simulink model "BmrTests"  (R2020a)
settings: Solver=FixedStepDiscrete  StartTime=0.0  StopTime=inf  FixedStep=Ts  RelTol=1e-3  EnableMultiTasking=on
undefined symbols (not defined in the file): BMR, DiscIntNeverNeededParam, MSR_REQUEST
libraries: simulink x2
settings Model: Creator=tbria  LastModifiedBy=Harjot
settings OptimizationCC: LifeSpan=inf
settings DebuggingCC: SFUnexpectedBacktrackingDiag=warning  SFNoUnconditionalDefaultTransitionDiag=warning  SFExecutionAtInitializationDiag=none  ArithmeticOperatorsInVariantConditions=warning
settings SFSimCC: SimUseLocalCustomCode=off  CustomCodeUndefinedFunction=UseInterfaceOnly
settings RTWCC: RTWUseLocalCustomCode=off
settings CodeAppCC: StateflowObjectComments=on
settings GRTTargetCC: TargetLangStandard=C89/C90 (ANSI)
settings ConfigComp: CovMetricSettings=dw  CovHtmlReporting=on  CovSaveCumulativeToWorkspaceVar=on  CovSaveSingleToWorkspaceVar=on  CovExternalEMLEnable=off

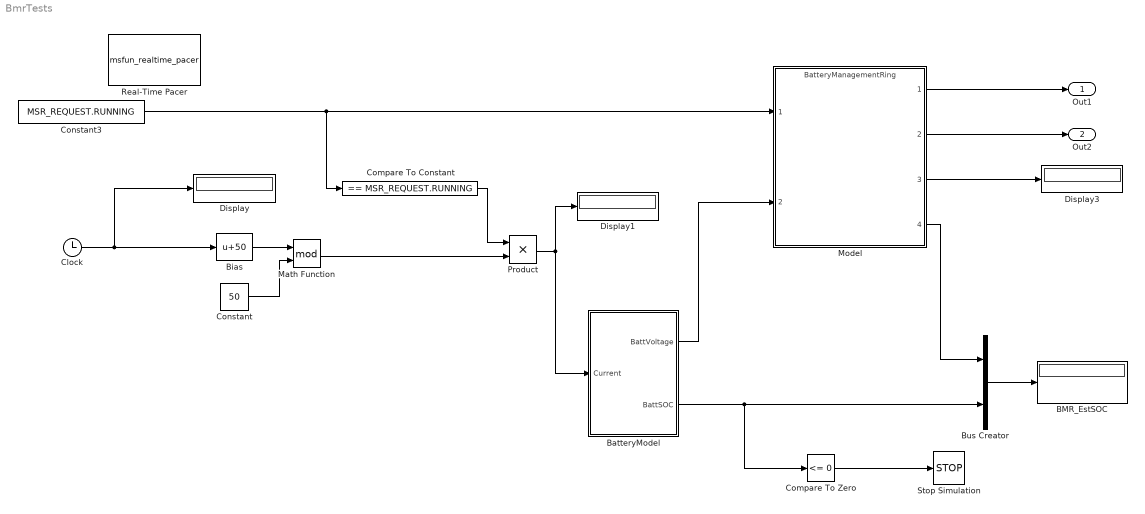
== system BmrTests ==
  BMR_EstSOC : Display
  BatteryModel : Subsystem
  Bias : Bias  Bias=50
  Bus Creator : BusCreator  Inputs=2
  Clock : Clock
  Compare To Constant : simulink/Logic and Bit Operations/Compare To Constant  relop===  const=MSR_REQUEST.RUNNING  OutDataTypeStr=boolean
  Compare To Zero : simulink/Logic and Bit Operations/Compare To Zero  relop=<=  OutDataTypeStr=boolean
  Constant : Constant  Value=50
  Constant3 : Constant  Value=MSR_REQUEST.RUNNING
  Display : Display
  Display1 : Display
  Display3 : Display
  Math Function : Math  Operator=mod  SignedPower=on  SaturateOnIntegerOverflow=on
  Model : ModelReference  ModelNameDialog=BatteryManagementRing.slx  SimulationMode=Normal  ModelReferenceVersion=1.56
  Product : Product
  Real-Time Pacer : M-S-Function  FunctionName=msfun_realtime_pacer  Parameters=simTimePerRealTime  mask(RealTime_Pacer){simTimePerRealTime=1}
      mask prompts: simTimePerRealTime "Speedup (Simulation Time / Real Time):"
      mask help:
      | Slow down a simulation to track real (i.e., wall clock) elapsed time.
      |
      | "Speedup" specifies the ratio between simulation time and real time
      | • Speedup = N => N sec. of simulation time per sec. of real time
      | • Speedup can be fractional (e.g., 0.5, 1.3).
      | • Speedup = inf => allow simulation to run at full speed
      |
      | Click on the Help button for details.
      mask Help: web('realtime_pacer_help.html', '-helpbrowser')
      mask Display: fprintf('Real-Time Pacer\nSpeedup = %g', simTimePerRealTime)
  Stop Simulation : Stop
  Out1 : Outport  VectorParamsAs1DForOutWhenUnconnected=off
  Out2 : Outport  Port=2  VectorParamsAs1DForOutWhenUnconnected=off
  wires:
  Model/3 -> Display3/1
  BatteryModel/1(BattVoltage) -> Model/2
  Bus Creator/1 -> BMR_EstSOC/1
  Model/4 -> Bus Creator/1
  Compare To Constant/1 -> Product/1
  Product/1 -> Display1/1, BatteryModel/1(Current)
  Clock/1 -> Display/1, Bias/1
  Constant/1 -> Math Function/2
  BatteryModel/2(BattSOC) -> Compare To Zero/1, Bus Creator/2
  Bias/1 -> Math Function/1
  Compare To Zero/1 -> Stop Simulation/1
  Model/1 -> Out1/1
  Model/2 -> Out2/1
  Constant3/1 -> Compare To Constant/1, Model/1
  Math Function/1 -> Product/2

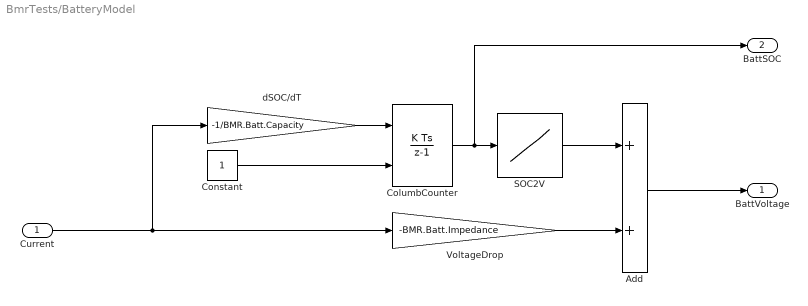
== system BmrTests/BatteryModel ==
  Current : Inport
  Add : Sum
  ColumbCounter : DiscreteIntegrator  InitialConditionSource=external  SampleTime=-1  ICPrevOutput=DiscIntNeverNeededParam  ICPrevScaledInput=DiscIntNeverNeededParam
  Constant : Constant
  SOC2V : Lookup_n-D  NumberOfTableDimensions=1  BreakpointsForDimension1=BMR.Batt.SOC.SOC  Table=BMR.Batt.SOC.Voltage  InternalRulePriority=Speed  RndMeth=Simplest  InputSameDT=on
  VoltageDrop : Gain  Gain=-BMR.Batt.Impedance
  dSOC/dT : Gain  Gain=-1/BMR.Batt.Capacity
  BattVoltage : Outport  VectorParamsAs1DForOutWhenUnconnected=off
  BattSOC : Outport  Port=2  VectorParamsAs1DForOutWhenUnconnected=off
  wires:
  Current/1 -> dSOC/dT/1, VoltageDrop/1
  dSOC/dT/1 -> ColumbCounter/1
  Constant/1 -> ColumbCounter/2
  ColumbCounter/1 -> BattSOC/1, SOC2V/1
  SOC2V/1 -> Add/1
  VoltageDrop/1 -> Add/2
  Add/1 -> BattVoltage/1
